simulink model "iot_casestudy_1_16"  (R2023a)
settings: Solver=VariableStepAuto  StartTime=0.0  StopTime=3.0  RelTol=1e-3
undefined symbols (not defined in the file or in its folder): m, n
(part 2 of 2)

== stateflow chart iot_casestudy_1_16/CameraDriver13 ==
  settings: updateMethod=CONTINUOUS
  state Operation
    state CarVisibility [parallel]
      settings: executionOrder=1
      state NoCar
        entry: car=0;
      state Car
        entry: car=1;
      (default) -> NoCar
      NoCar -> Car : [traffic_state==1]
      Car -> NoCar : [traffic_state==0]
    state DriverOperation [parallel]
      settings: executionOrder=2
      state Main
      (default) -> Main : {i=1;}
      Main -> (junction 22) : schedule
          | [image_request]
      (junction 22) -> Main [order 1] : [(car==1)&&(blurryness(i)==1)]
          | {image.data=1;send(image);i = i + 1;}
      (junction 22) -> Main [order 2] : {image.data=0;
          | send(image);i = i + 1;}
  data: image_request input; traffic_state input; blurryness input; image output; car local; i local; schedule input

== stateflow chart iot_casestudy_1_16/CameraDriver14 ==
  settings: updateMethod=CONTINUOUS
  state Operation
    state CarVisibility [parallel]
      settings: executionOrder=1
      state NoCar
        entry: car=0;
      state Car
        entry: car=1;
      (default) -> NoCar
      NoCar -> Car : [traffic_state==1]
      Car -> NoCar : [traffic_state==0]
    state DriverOperation [parallel]
      settings: executionOrder=2
      state Main
      (default) -> Main : {i=1;}
      Main -> (junction 22) : schedule[image_request]
      (junction 22) -> Main [order 2] : {image.data=0;
          | send(image);i = i + 1;}
      (junction 22) -> Main [order 1] : [(car==1)&&(blurryness(i)==1)]
          | {image.data=1;i = i + 1;send(image);}
  data: image_request input; traffic_state input; blurryness input; image output; car local; i local; schedule input

== stateflow chart iot_casestudy_1_16/CameraDriver15 ==
  settings: updateMethod=CONTINUOUS
  state Operation
    state CarVisibility [parallel]
      settings: executionOrder=1
      state NoCar
        entry: car=0;
      state Car
        entry: car=1;
      (default) -> NoCar
      NoCar -> Car : [traffic_state==1]
      Car -> NoCar : [traffic_state==0]
    state DriverOperation [parallel]
      settings: executionOrder=2
      state Main
      (default) -> Main : {i=1;}
      Main -> (junction 22) : schedule
          | [image_request]
      (junction 22) -> Main [order 1] : [(car==1)&&(blurryness(i)==1)]
          | {image.data=1;send(image);i = i + 1;}
      (junction 22) -> Main [order 2] : {image.data=0;
          | send(image);i = i + 1;}
  data: image_request input; traffic_state input; blurryness input; image output; car local; i local; schedule input

== stateflow chart iot_casestudy_1_16/CameraDriver8 ==
  settings: updateMethod=CONTINUOUS
  state Operation
    state CarVisibility [parallel]
      settings: executionOrder=1
      state NoCar
        entry: car=0;
      state Car
        entry: car=1;
      (default) -> NoCar
      NoCar -> Car : [traffic_state==1]
      Car -> NoCar : [traffic_state==0]
    state DriverOperation [parallel]
      settings: executionOrder=2
      state Main
      (default) -> Main : {i=1;}
      Main -> (junction 22) : schedule[image_request]
      (junction 22) -> Main [order 2] : {image.data=0;
          | send(image);i = i + 1;}
      (junction 22) -> Main [order 1] : [(car==1)&&(blurryness(i)==1)]
          | {image.data=1;i = i + 1;send(image);}
  data: image_request input; traffic_state input; blurryness input; image output; car local; i local; schedule input

== stateflow chart iot_casestudy_1_16/CameraDriver9 ==
  settings: updateMethod=CONTINUOUS
  state Operation
    state CarVisibility [parallel]
      settings: executionOrder=1
      state NoCar
        entry: car=0;
      state Car
        entry: car=1;
      (default) -> NoCar
      NoCar -> Car : [traffic_state==1]
      Car -> NoCar : [traffic_state==0]
    state DriverOperation [parallel]
      settings: executionOrder=2
      state Main
      (default) -> Main : {i=1;}
      Main -> (junction 22) : schedule
          | [image_request]
      (junction 22) -> Main [order 1] : [(car==1)&&(blurryness(i)==1)]
          | {image.data=1;send(image);i = i + 1;}
      (junction 22) -> Main [order 2] : {image.data=0;
          | send(image);i = i + 1;}
  data: image_request input; traffic_state input; blurryness input; image output; car local; i local; schedule input

== stateflow chart iot_casestudy_1_16/CameraScheduler10 ==
  settings: updateMethod=CONTINUOUS  executeAtInitialization=1
  state Main
    entry:
    dt=timer_array[i];
  (default) -> Main : {i=1;dt=0;}
  Main -> Main : after(dt,msec){i=i+1;send(schedule_driver);send(schedule_control);}
  data: timer_array input; schedule_driver output double; schedule_control output double; dt local double; dt2 local double; i local double =0.0

== stateflow chart iot_casestudy_1_16/CameraScheduler11 ==
  settings: updateMethod=CONTINUOUS  executeAtInitialization=1
  state Main
    entry:
    dt=timer_array[i];
  (default) -> Main : {i=0;dt=0;}
  Main -> Main : after(dt,msec){i=i+1;send(schedule_driver);send(schedule_control);}
  data: timer_array input; i local double; schedule_driver output double; schedule_control output double; dt local double

== stateflow chart iot_casestudy_1_16/CameraScheduler12 ==
  settings: updateMethod=CONTINUOUS  executeAtInitialization=1
  state Main
    entry:
    dt=timer_array[i];
  (default) -> Main : {i=1;dt=0;}
  Main -> Main : after(dt,msec){i=i+1;send(schedule_driver);send(schedule_control);}
  data: timer_array input; schedule_driver output double; schedule_control output double; dt local double; dt2 local double; i local double =0.0

== stateflow chart iot_casestudy_1_16/CameraScheduler13 ==
  settings: updateMethod=CONTINUOUS  executeAtInitialization=1
  state Main
    entry:
    dt=timer_array[i];
  (default) -> Main : {i=0;dt=0;}
  Main -> Main : after(dt,msec){i=i+1;send(schedule_driver);send(schedule_control);}
  data: timer_array input; i local double; schedule_driver output double; schedule_control output double; dt local double

== stateflow chart iot_casestudy_1_16/CameraScheduler14 ==
  settings: updateMethod=CONTINUOUS  executeAtInitialization=1
  state Main
    entry:
    dt=timer_array[i];
  (default) -> Main : {i=1;dt=0;}
  Main -> Main : after(dt,msec){i=i+1;send(schedule_driver);send(schedule_control);}
  data: timer_array input; schedule_driver output double; schedule_control output double; dt local double; dt2 local double; i local double =0.0

== stateflow chart iot_casestudy_1_16/CameraScheduler15 ==
  settings: updateMethod=CONTINUOUS  executeAtInitialization=1
  state Main
    entry:
    dt=timer_array[i];
  (default) -> Main : {i=0;dt=0;}
  Main -> Main : after(dt,msec){i=i+1;send(schedule_driver);send(schedule_control);}
  data: timer_array input; i local double; schedule_driver output double; schedule_control output double; dt local double

== stateflow chart iot_casestudy_1_16/CameraScheduler8 ==
  settings: updateMethod=CONTINUOUS  executeAtInitialization=1
  state Main
    entry:
    dt=timer_array[i];
  (default) -> Main : {i=1;dt=0;}
  Main -> Main : after(dt,msec){i=i+1;send(schedule_driver);send(schedule_control);}
  data: timer_array input; schedule_driver output double; schedule_control output double; dt local double; dt2 local double; i local double =0.0

== stateflow chart iot_casestudy_1_16/CameraScheduler9 ==
  settings: updateMethod=CONTINUOUS  executeAtInitialization=1
  state Main
    entry:
    dt=timer_array[i];
  (default) -> Main : {i=0;dt=0;}
  Main -> Main : after(dt,msec){i=i+1;send(schedule_driver);send(schedule_control);}
  data: timer_array input; i local double; schedule_driver output double; schedule_control output double; dt local double

== stateflow chart iot_casestudy_1_16/CameraDriver ==
  settings: updateMethod=CONTINUOUS
  state Operation
    state CarVisibility [parallel]
      settings: executionOrder=1
      state NoCar
        entry: car=0;
      state Car
        entry: car=1;
      (default) -> NoCar
      NoCar -> Car : [traffic_state==1]
      Car -> NoCar : [traffic_state==0]
    state DriverOperation [parallel]
      settings: executionOrder=2
      state Main
      (default) -> Main : {i=1;}
      Main -> (junction 22) : schedule[image_request]
      (junction 22) -> Main [order 2] : {image.data=0;
          | send(image);i = i + 1;}
      (junction 22) -> Main [order 1] : [(car==1)&&(blurryness(i)==1)]
          | {image.data=1;i = i + 1;send(image);}
  data: image_request input; traffic_state input; blurryness input; image output; car local; i local; schedule input

== stateflow chart iot_casestudy_1_16/CameraControl ==
  settings: updateMethod=CONTINUOUS
  state Operation
    state RequestHangling [parallel]
      settings: executionOrder=1
      state Operation1
      (default) -> Operation1 : {image_request=1;}
      Operation1 -> Operation1 : schedule{image_request=1;}
    state ImageMessaging [parallel]
      settings: executionOrder=2
      state Operation2
        entry:
        validity=isvalid(imageIn);
      (default) -> Operation2 : {i=1;}
      (junction 28) -> Operation2 [order 1] : [validity==1]
          | {receive(imageIn);i = i + 1;
          | imageOut.data=imageIn.data
          | send(imageOut);}
      (junction 28) -> Operation2 [order 2] : {i = i + 1;receive(imageIn);}
      (junction 19) -> (junction 28) [order 1] : [network_faults(i)==0]
      (junction 19) -> Operation2 [order 2] : {receive(imageIn);i = i + 1;}
      Operation2 -> (junction 19) : schedule
  (default) -> Operation
  data: image_request output; imageIn input; i local; network_faults input; imageOut output; schedule input; validity local

== stateflow chart iot_casestudy_1_16/Traffic ==
  settings: updateMethod=CONTINUOUS
  state Nocar
    entry:
    traffic_state=0;
  state Car
    entry:
    traffic_state=1;
  state Nocar1
    entry:
    traffic_state=0;
  (default) -> Nocar
  Nocar -> Car : after(arrive_time,msec)
  Car -> Nocar1 : after(visibility_time,msec)
  data: arrive_time input; visibility_time input; traffic_state output

== stateflow chart iot_casestudy_1_16/Edge ==
  state Waiting
  state NotRecognized
    wait_time=elapsed(msec);
  state Recognized
  (default) -> Waiting : {faults=0;}
  Waiting -> Waiting [order 2] : image2{receive(image2);}
  Waiting -> Waiting [order 7] : image5{receive(image5);}
  Waiting -> Waiting [order 8] : image7{receive(image7);}
  Waiting -> Waiting [order 5] : image3{receive(image3);}
  Waiting -> Waiting [order 9] : image8{receive(image8);}
  Waiting -> Waiting [order 6] : image4{receive(image4);}
  Waiting -> Waiting [order 3] : image1{receive(image1);}
  Waiting -> Waiting [order 1] : image6{receive(image6);}
  Waiting -> NotRecognized [order 4] : [traffic_state==1]
  NotRecognized -> Waiting [order 1] : [traffic_state==0]
      | {faults=1;}
  Recognized -> Waiting [order 1] : [traffic_state==0]
  Waiting -> Waiting [order 10] : image9{receive(image9);}
  Waiting -> Waiting [order 11] : image10{receive(image10);}
  Waiting -> Waiting [order 12] : image11{receive(image11);}
  Waiting -> Waiting [order 13] : image12{receive(image12);}
  Waiting -> Waiting [order 14] : image13{receive(image13);}
  Waiting -> Waiting [order 15] : image14{receive(image14);}
  Waiting -> Waiting [order 16] : image15{receive(image15);}
  Waiting -> Waiting [order 17] : image16{receive(image16);}
  (junction 119) -> NotRecognized [order 2]
  NotRecognized -> (junction 119) [order 3] : image16
      | {receive(image16);}
  (junction 117) -> NotRecognized [order 2]
  NotRecognized -> (junction 117) [order 4] : image15
      | {receive(image15);}
  (junction 106) -> NotRecognized [order 2]
  NotRecognized -> (junction 106) [order 5] : image14
      | {receive(image14);}
  (junction 132) -> NotRecognized [order 2]
  NotRecognized -> (junction 132) [order 6] : image13
      | {receive(image13);}
  (junction 108) -> NotRecognized [order 2]
  NotRecognized -> (junction 108) [order 7] : image12
      | {receive(image12);}
  (junction 113) -> NotRecognized [order 2]
  NotRecognized -> (junction 113) [order 8] : image11
      | {receive(image11);}
  (junction 105) -> NotRecognized [order 2]
  NotRecognized -> (junction 105) [order 9] : image10
      | {receive(image10);}
  (junction 120) -> NotRecognized [order 2]
  NotRecognized -> (junction 120) [order 11] : image9
      | {receive(image9);}
  (junction 64) -> NotRecognized [order 2]
  NotRecognized -> (junction 64) [order 17] : image8
      | {receive(image8);}
  (junction 63) -> NotRecognized [order 2]
  NotRecognized -> (junction 63) [order 16] : image7
      | {receive(image7);}
  (junction 62) -> NotRecognized [order 2]
  NotRecognized -> (junction 62) [order 15] : image6
      | {receive(image6);}
  (junction 61) -> NotRecognized [order 2]
  NotRecognized -> (junction 61) [order 14] : image5
      | {receive(image5);}
  (junction 49) -> NotRecognized [order 2]
  NotRecognized -> (junction 49) [order 13] : image4
      | {receive(image4);}
  (junction 45) -> NotRecognized [order 2]
  NotRecognized -> (junction 45) [order 12] : image3
      | {receive(image3);}
  (junction 22) -> NotRecognized [order 2]
  NotRecognized -> (junction 22) [order 2] : image2
      | {receive(image2);}
  (junction 10) -> NotRecognized [order 2]
  NotRecognized -> (junction 10) [order 10] : image1{receive(image1);}
  (junction 49) -> Recognized [order 1] : [image4.data==1]
  (junction 22) -> Recognized [order 1] : [image2.data==1]
  (junction 105) -> Recognized [order 1] : [image10.data==1]
  (junction 64) -> Recognized [order 1] : [image8.data==1]
  (junction 62) -> Recognized [order 1] : [image6.data==1]
  (junction 119) -> Recognized [order 1] : [image16.data==1]
  (junction 106) -> Recognized [order 1] : [image14.data==1]
  (junction 108) -> Recognized [order 1] : [image12.data==1]
  (junction 132) -> Recognized [order 1] : [image13.data==1]
  (junction 113) -> Recognized [order 1] : [image11.data==1]
  (junction 120) -> Recognized [order 1] : [image9.data==1]
  (junction 63) -> Recognized [order 1] : [image7.data==1]
  (junction 61) -> Recognized [order 1] : [image5.data==1]
  (junction 117) -> Recognized [order 1] : [image15.data==1]
  (junction 45) -> Recognized [order 1] : [image3.data==1]
  (junction 10) -> Recognized [order 1] : [image1.data==1]
  Recognized -> Recognized [order 10] : image9{receive(image9);}
  Recognized -> Recognized [order 11] : image10{receive(image10);}
  Recognized -> Recognized [order 12] : image11{receive(image11);}
  Recognized -> Recognized [order 13] : image12{receive(image12);}
  Recognized -> Recognized [order 14] : image13{receive(image13);}
  Recognized -> Recognized [order 15] : image14{receive(image14);}
  Recognized -> Recognized [order 16] : image15{receive(image15);}
  Recognized -> Recognized [order 17] : image16{receive(image16);}
  Recognized -> Recognized [order 6] : image8{receive(image8);}
  Recognized -> Recognized [order 7] : image7{receive(image7);}
  Recognized -> Recognized [order 8] : image6{receive(image6);}
  Recognized -> Recognized [order 9] : image5{receive(image5);}
  Recognized -> Recognized [order 2] : image3{receive(image3);}
  Recognized -> Recognized [order 5] : image4{receive(image4);}
  Recognized -> Recognized [order 3] : image2{receive(image2);}
  Recognized -> Recognized [order 4] : image1{receive(image1);}
  data: traffic_state input; image1 input; faults output; image2 input; wait_time output; image3 input; image4 input; image5 input; image6 input; image7 input; image8 input; image9 input; image10 input; image11 input; image12 input; image13 input; image14 input; image15 input; image16 input

== stateflow chart iot_casestudy_1_16/CameraScheduler ==
  settings: updateMethod=CONTINUOUS  executeAtInitialization=1
  state Main
    entry:
    dt=timer_array[i];
  (default) -> Main : {i=1;dt=0;}
  Main -> Main : after(dt,msec){i=i+1;send(schedule_driver);send(schedule_control);}
  data: timer_array input; schedule_driver output double; schedule_control output double; dt local double; dt2 local double; i output double =0.0

== stateflow chart iot_casestudy_1_16/CameraControl1 ==
  settings: updateMethod=CONTINUOUS
  state Operation
    state RequestHangling [parallel]
      settings: executionOrder=1
      note: {image_request=1;}
      state Operation1
      (default) -> Operation1
      Operation1 -> Operation1 : schedule{image_request=1;}
    state ImageMessaging [parallel]
      settings: executionOrder=2
      state Operation2
        entry:
        validity=isvalid(imageIn);
      (default) -> Operation2 : {i=1;}
      (junction 29) -> Operation2 [order 1] : [isvalid(imageIn)==1]
          | {receive(imageIn);i = i + 1;
          | imageOut.data=imageIn.data;
          | send(imageOut);}
      (junction 19) -> Operation2 [order 2] : {receive(imageIn);i = i + 1;}
      Operation2 -> (junction 19) : schedule
      (junction 29) -> Operation2 [order 2] : {i = i + 1;receive(imageIn);}
      (junction 19) -> (junction 29) [order 1] : [network_faults(i)==0]
  (default) -> Operation
  data: image_request output; imageIn input; i local; network_faults input; imageOut output; schedule input; validity local

== stateflow chart iot_casestudy_1_16/CameraDriver1 ==
  settings: updateMethod=CONTINUOUS
  state Operation
    state CarVisibility [parallel]
      settings: executionOrder=1
      state NoCar
        entry: car=0;
      state Car
        entry: car=1;
      (default) -> NoCar
      NoCar -> Car : [traffic_state==1]
      Car -> NoCar : [traffic_state==0]
    state DriverOperation [parallel]
      settings: executionOrder=2
      state Main
      (default) -> Main : {i=1;}
      Main -> (junction 22) : schedule
          | [image_request]
      (junction 22) -> Main [order 1] : [(car==1)&&(blurryness(i)==1)]
          | {image.data=1;send(image);i = i + 1;}
      (junction 22) -> Main [order 2] : {image.data=0;
          | send(image);i = i + 1;}
  data: image_request input; traffic_state input; blurryness input; image output; car local; i local; schedule input

== stateflow chart iot_casestudy_1_16/CameraScheduler1 ==
  settings: updateMethod=CONTINUOUS  executeAtInitialization=1
  state Main
    entry:
    dt=timer_array[i];
  (default) -> Main : {i=0;dt=0;}
  Main -> Main : after(dt,msec){i=i+1;send(schedule_driver);send(schedule_control);}
  data: timer_array input; i local double; schedule_driver output double; schedule_control output double; dt local double

== stateflow chart iot_casestudy_1_16/CameraControl2 ==
  settings: updateMethod=CONTINUOUS
  state Operation
    state RequestHangling [parallel]
      settings: executionOrder=1
      state Operation1
      (default) -> Operation1 : {image_request=1;}
      Operation1 -> Operation1 : schedule{image_request=1;}
    state ImageMessaging [parallel]
      settings: executionOrder=2
      state Operation2
        entry:
        validity=isvalid(imageIn);
      (default) -> Operation2 : {i=1;}
      (junction 28) -> Operation2 [order 1] : [validity==1]
          | {receive(imageIn);i = i + 1;
          | imageOut.data=imageIn.data
          | send(imageOut);}
      (junction 28) -> Operation2 [order 2] : {i = i + 1;receive(imageIn);}
      (junction 19) -> (junction 28) [order 1] : [network_faults(i)==0]
      (junction 19) -> Operation2 [order 2] : {receive(imageIn);i = i + 1;}
      Operation2 -> (junction 19) : schedule
  (default) -> Operation
  data: image_request output; imageIn input; i local; network_faults input; imageOut output; schedule input; validity local

== stateflow chart iot_casestudy_1_16/CameraControl3 ==
  settings: updateMethod=CONTINUOUS
  state Operation
    state RequestHangling [parallel]
      settings: executionOrder=1
      note: {image_request=1;}
      state Operation1
      (default) -> Operation1
      Operation1 -> Operation1 : schedule{image_request=1;}
    state ImageMessaging [parallel]
      settings: executionOrder=2
      state Operation2
        entry:
        validity=isvalid(imageIn);
      (default) -> Operation2 : {i=1;}
      (junction 29) -> Operation2 [order 1] : [isvalid(imageIn)==1]
          | {receive(imageIn);i = i + 1;
          | imageOut.data=imageIn.data;
          | send(imageOut);}
      (junction 19) -> Operation2 [order 2] : {receive(imageIn);i = i + 1;}
      Operation2 -> (junction 19) : schedule
      (junction 29) -> Operation2 [order 2] : {i = i + 1;receive(imageIn);}
      (junction 19) -> (junction 29) [order 1] : [network_faults(i)==0]
  (default) -> Operation
  data: image_request output; imageIn input; i local; network_faults input; imageOut output; schedule input; validity local

== stateflow chart iot_casestudy_1_16/CameraDriver2 ==
  settings: updateMethod=CONTINUOUS
  state Operation
    state CarVisibility [parallel]
      settings: executionOrder=1
      state NoCar
        entry: car=0;
      state Car
        entry: car=1;
      (default) -> NoCar
      NoCar -> Car : [traffic_state==1]
      Car -> NoCar : [traffic_state==0]
    state DriverOperation [parallel]
      settings: executionOrder=2
      state Main
      (default) -> Main : {i=1;}
      Main -> (junction 22) : schedule[image_request]
      (junction 22) -> Main [order 2] : {image.data=0;
          | send(image);i = i + 1;}
      (junction 22) -> Main [order 1] : [(car==1)&&(blurryness(i)==1)]
          | {image.data=1;i = i + 1;send(image);}
  data: image_request input; traffic_state input; blurryness input; image output; car local; i local; schedule input

== stateflow chart iot_casestudy_1_16/CameraDriver3 ==
  settings: updateMethod=CONTINUOUS
  state Operation
    state CarVisibility [parallel]
      settings: executionOrder=1
      state NoCar
        entry: car=0;
      state Car
        entry: car=1;
      (default) -> NoCar
      NoCar -> Car : [traffic_state==1]
      Car -> NoCar : [traffic_state==0]
    state DriverOperation [parallel]
      settings: executionOrder=2
      state Main
      (default) -> Main : {i=1;}
      Main -> (junction 22) : schedule
          | [image_request]
      (junction 22) -> Main [order 1] : [(car==1)&&(blurryness(i)==1)]
          | {image.data=1;send(image);i = i + 1;}
      (junction 22) -> Main [order 2] : {image.data=0;
          | send(image);i = i + 1;}
  data: image_request input; traffic_state input; blurryness input; image output; car local; i local; schedule input

== stateflow chart iot_casestudy_1_16/CameraScheduler2 ==
  settings: updateMethod=CONTINUOUS  executeAtInitialization=1
  state Main
    entry:
    dt=timer_array[i];
  (default) -> Main : {i=1;dt=0;}
  Main -> Main : after(dt,msec){i=i+1;send(schedule_driver);send(schedule_control);}
  data: timer_array input; schedule_driver output double; schedule_control output double; dt local double; dt2 local double; i output double =0.0

== stateflow chart iot_casestudy_1_16/CameraScheduler3 ==
  settings: updateMethod=CONTINUOUS  executeAtInitialization=1
  state Main
    entry:
    dt=timer_array[i];
  (default) -> Main : {i=0;dt=0;}
  Main -> Main : after(dt,msec){i=i+1;send(schedule_driver);send(schedule_control);}
  data: timer_array input; i local double; schedule_driver output double; schedule_control output double; dt local double

== stateflow chart iot_casestudy_1_16/CameraControl4 ==
  settings: updateMethod=CONTINUOUS
  state Operation
    state RequestHangling [parallel]
      settings: executionOrder=1
      state Operation1
      (default) -> Operation1 : {image_request=1;}
      Operation1 -> Operation1 : schedule{image_request=1;}
    state ImageMessaging [parallel]
      settings: executionOrder=2
      state Operation2
        entry:
        validity=isvalid(imageIn);
      (default) -> Operation2 : {i=1;}
      (junction 28) -> Operation2 [order 1] : [validity==1]
          | {receive(imageIn);i = i + 1;
          | imageOut.data=imageIn.data
          | send(imageOut);}
      (junction 28) -> Operation2 [order 2] : {i = i + 1;receive(imageIn);}
      (junction 19) -> (junction 28) [order 1] : [network_faults(i)==0]
      (junction 19) -> Operation2 [order 2] : {receive(imageIn);i = i + 1;}
      Operation2 -> (junction 19) : schedule
  (default) -> Operation
  data: image_request output; imageIn input; i local; network_faults input; imageOut output; schedule input; validity local

== stateflow chart iot_casestudy_1_16/CameraControl5 ==
  settings: updateMethod=CONTINUOUS
  state Operation
    state RequestHangling [parallel]
      settings: executionOrder=1
      note: {image_request=1;}
      state Operation1
      (default) -> Operation1
      Operation1 -> Operation1 : schedule{image_request=1;}
    state ImageMessaging [parallel]
      settings: executionOrder=2
      state Operation2
        entry:
        validity=isvalid(imageIn);
      (default) -> Operation2 : {i=1;}
      (junction 29) -> Operation2 [order 1] : [isvalid(imageIn)==1]
          | {receive(imageIn);i = i + 1;
          | imageOut.data=imageIn.data;
          | send(imageOut);}
      (junction 19) -> Operation2 [order 2] : {receive(imageIn);i = i + 1;}
      Operation2 -> (junction 19) : schedule
      (junction 29) -> Operation2 [order 2] : {i = i + 1;receive(imageIn);}
      (junction 19) -> (junction 29) [order 1] : [network_faults(i)==0]
  (default) -> Operation
  data: image_request output; imageIn input; i local; network_faults input; imageOut output; schedule input; validity local

== stateflow chart iot_casestudy_1_16/CameraControl6 ==
  settings: updateMethod=CONTINUOUS
  state Operation
    state RequestHangling [parallel]
      settings: executionOrder=1
      state Operation1
      (default) -> Operation1 : {image_request=1;}
      Operation1 -> Operation1 : schedule{image_request=1;}
    state ImageMessaging [parallel]
      settings: executionOrder=2
      state Operation2
        entry:
        validity=isvalid(imageIn);
      (default) -> Operation2 : {i=1;}
      (junction 28) -> Operation2 [order 1] : [validity==1]
          | {receive(imageIn);i = i + 1;
          | imageOut.data=imageIn.data
          | send(imageOut);}
      (junction 28) -> Operation2 [order 2] : {i = i + 1;receive(imageIn);}
      (junction 19) -> (junction 28) [order 1] : [network_faults(i)==0]
      (junction 19) -> Operation2 [order 2] : {receive(imageIn);i = i + 1;}
      Operation2 -> (junction 19) : schedule
  (default) -> Operation
  data: image_request output; imageIn input; i local; network_faults input; imageOut output; schedule input; validity local

== stateflow chart iot_casestudy_1_16/CameraControl7 ==
  settings: updateMethod=CONTINUOUS
  state Operation
    state RequestHangling [parallel]
      settings: executionOrder=1
      note: {image_request=1;}
      state Operation1
      (default) -> Operation1
      Operation1 -> Operation1 : schedule{image_request=1;}
    state ImageMessaging [parallel]
      settings: executionOrder=2
      state Operation2
        entry:
        validity=isvalid(imageIn);
      (default) -> Operation2 : {i=1;}
      (junction 29) -> Operation2 [order 1] : [isvalid(imageIn)==1]
          | {receive(imageIn);i = i + 1;
          | imageOut.data=imageIn.data;
          | send(imageOut);}
      (junction 19) -> Operation2 [order 2] : {receive(imageIn);i = i + 1;}
      Operation2 -> (junction 19) : schedule
      (junction 29) -> Operation2 [order 2] : {i = i + 1;receive(imageIn);}
      (junction 19) -> (junction 29) [order 1] : [network_faults(i)==0]
  (default) -> Operation
  data: image_request output; imageIn input; i local; network_faults input; imageOut output; schedule input; validity local

== stateflow chart iot_casestudy_1_16/CameraDriver4 ==
  settings: updateMethod=CONTINUOUS
  state Operation
    state CarVisibility [parallel]
      settings: executionOrder=1
      state NoCar
        entry: car=0;
      state Car
        entry: car=1;
      (default) -> NoCar
      NoCar -> Car : [traffic_state==1]
      Car -> NoCar : [traffic_state==0]
    state DriverOperation [parallel]
      settings: executionOrder=2
      state Main
      (default) -> Main : {i=1;}
      Main -> (junction 22) : schedule[image_request]
      (junction 22) -> Main [order 2] : {image.data=0;
          | send(image);i = i + 1;}
      (junction 22) -> Main [order 1] : [(car==1)&&(blurryness(i)==1)]
          | {image.data=1;i = i + 1;send(image);}
  data: image_request input; traffic_state input; blurryness input; image output; car local; i local; schedule input

== stateflow chart iot_casestudy_1_16/CameraDriver5 ==
  settings: updateMethod=CONTINUOUS
  state Operation
    state CarVisibility [parallel]
      settings: executionOrder=1
      state NoCar
        entry: car=0;
      state Car
        entry: car=1;
      (default) -> NoCar
      NoCar -> Car : [traffic_state==1]
      Car -> NoCar : [traffic_state==0]
    state DriverOperation [parallel]
      settings: executionOrder=2
      state Main
      (default) -> Main : {i=1;}
      Main -> (junction 22) : schedule
          | [image_request]
      (junction 22) -> Main [order 1] : [(car==1)&&(blurryness(i)==1)]
          | {image.data=1;send(image);i = i + 1;}
      (junction 22) -> Main [order 2] : {image.data=0;
          | send(image);i = i + 1;}
  data: image_request input; traffic_state input; blurryness input; image output; car local; i local; schedule input

== stateflow chart iot_casestudy_1_16/CameraDriver6 ==
  settings: updateMethod=CONTINUOUS
  state Operation
    state CarVisibility [parallel]
      settings: executionOrder=1
      state NoCar
        entry: car=0;
      state Car
        entry: car=1;
      (default) -> NoCar
      NoCar -> Car : [traffic_state==1]
      Car -> NoCar : [traffic_state==0]
    state DriverOperation [parallel]
      settings: executionOrder=2
      state Main
      (default) -> Main : {i=1;}
      Main -> (junction 22) : schedule[image_request]
      (junction 22) -> Main [order 2] : {image.data=0;
          | send(image);i = i + 1;}
      (junction 22) -> Main [order 1] : [(car==1)&&(blurryness(i)==1)]
          | {image.data=1;i = i + 1;send(image);}
  data: image_request input; traffic_state input; blurryness input; image output; car local; i local; schedule input

== stateflow chart iot_casestudy_1_16/CameraDriver7 ==
  settings: updateMethod=CONTINUOUS
  state Operation
    state CarVisibility [parallel]
      settings: executionOrder=1
      state NoCar
        entry: car=0;
      state Car
        entry: car=1;
      (default) -> NoCar
      NoCar -> Car : [traffic_state==1]
      Car -> NoCar : [traffic_state==0]
    state DriverOperation [parallel]
      settings: executionOrder=2
      state Main
      (default) -> Main : {i=1;}
      Main -> (junction 22) : schedule
          | [image_request]
      (junction 22) -> Main [order 1] : [(car==1)&&(blurryness(i)==1)]
          | {image.data=1;send(image);i = i + 1;}
      (junction 22) -> Main [order 2] : {image.data=0;
          | send(image);i = i + 1;}
  data: image_request input; traffic_state input; blurryness input; image output; car local; i local; schedule input

== stateflow chart iot_casestudy_1_16/CameraScheduler4 ==
  settings: updateMethod=CONTINUOUS  executeAtInitialization=1
  state Main
    entry:
    dt=timer_array[i];
  (default) -> Main : {i=1;dt=0;}
  Main -> Main : after(dt,msec){i=i+1;send(schedule_driver);send(schedule_control);}
  data: timer_array input; schedule_driver output double; schedule_control output double; dt local double; dt2 local double; i output double =0.0

== stateflow chart iot_casestudy_1_16/CameraScheduler5 ==
  settings: updateMethod=CONTINUOUS  executeAtInitialization=1
  state Main
    entry:
    dt=timer_array[i];
  (default) -> Main : {i=0;dt=0;}
  Main -> Main : after(dt,msec){i=i+1;send(schedule_driver);send(schedule_control);}
  data: timer_array input; i local double; schedule_driver output double; schedule_control output double; dt local double

== stateflow chart iot_casestudy_1_16/CameraScheduler6 ==
  settings: updateMethod=CONTINUOUS  executeAtInitialization=1
  state Main
    entry:
    dt=timer_array[i];
  (default) -> Main : {i=1;dt=0;}
  Main -> Main : after(dt,msec){i=i+1;send(schedule_driver);send(schedule_control);}
  data: timer_array input; schedule_driver output double; schedule_control output double; dt local double; dt2 local double; i output double =0.0

== stateflow chart iot_casestudy_1_16/CameraScheduler7 ==
  settings: updateMethod=CONTINUOUS  executeAtInitialization=1
  state Main
    entry:
    dt=timer_array[i];
  (default) -> Main : {i=0;dt=0;}
  Main -> Main : after(dt,msec){i=i+1;send(schedule_driver);send(schedule_control);}
  data: timer_array input; i local double; schedule_driver output double; schedule_control output double; dt local double

== stateflow chart iot_casestudy_1_16/CameraControl10 ==
  settings: updateMethod=CONTINUOUS
  state Operation
    state RequestHangling [parallel]
      settings: executionOrder=1
      state Operation1
      (default) -> Operation1 : {image_request=1;}
      Operation1 -> Operation1 : schedule{image_request=1;}
    state ImageMessaging [parallel]
      settings: executionOrder=2
      state Operation2
        entry:
        validity=isvalid(imageIn);
      (default) -> Operation2 : {i=1;}
      (junction 28) -> Operation2 [order 1] : [validity==1]
          | {receive(imageIn);i = i + 1;
          | imageOut.data=imageIn.data
          | send(imageOut);}
      (junction 28) -> Operation2 [order 2] : {i = i + 1;receive(imageIn);}
      (junction 19) -> (junction 28) [order 1] : [network_faults(i)==0]
      (junction 19) -> Operation2 [order 2] : {receive(imageIn);i = i + 1;}
      Operation2 -> (junction 19) : schedule
  (default) -> Operation
  data: image_request output; imageIn input; i local; network_faults input; imageOut output; schedule input; validity local

== stateflow chart iot_casestudy_1_16/CameraControl11 ==
  settings: updateMethod=CONTINUOUS
  state Operation
    state RequestHangling [parallel]
      settings: executionOrder=1
      note: {image_request=1;}
      state Operation1
      (default) -> Operation1
      Operation1 -> Operation1 : schedule{image_request=1;}
    state ImageMessaging [parallel]
      settings: executionOrder=2
      state Operation2
        entry:
        validity=isvalid(imageIn);
      (default) -> Operation2 : {i=1;}
      (junction 29) -> Operation2 [order 1] : [isvalid(imageIn)==1]
          | {receive(imageIn);i = i + 1;
          | imageOut.data=imageIn.data;
          | send(imageOut);}
      (junction 19) -> Operation2 [order 2] : {receive(imageIn);i = i + 1;}
      Operation2 -> (junction 19) : schedule
      (junction 29) -> Operation2 [order 2] : {i = i + 1;receive(imageIn);}
      (junction 19) -> (junction 29) [order 1] : [network_faults(i)==0]
  (default) -> Operation
  data: image_request output; imageIn input; i local; network_faults input; imageOut output; schedule input; validity local

== stateflow chart iot_casestudy_1_16/CameraControl12 ==
  settings: updateMethod=CONTINUOUS
  state Operation
    state RequestHangling [parallel]
      settings: executionOrder=1
      state Operation1
      (default) -> Operation1 : {image_request=1;}
      Operation1 -> Operation1 : schedule{image_request=1;}
    state ImageMessaging [parallel]
      settings: executionOrder=2
      state Operation2
        entry:
        validity=isvalid(imageIn);
      (default) -> Operation2 : {i=1;}
      (junction 28) -> Operation2 [order 1] : [validity==1]
          | {receive(imageIn);i = i + 1;
          | imageOut.data=imageIn.data
          | send(imageOut);}
      (junction 28) -> Operation2 [order 2] : {i = i + 1;receive(imageIn);}
      (junction 19) -> (junction 28) [order 1] : [network_faults(i)==0]
      (junction 19) -> Operation2 [order 2] : {receive(imageIn);i = i + 1;}
      Operation2 -> (junction 19) : schedule
  (default) -> Operation
  data: image_request output; imageIn input; i local; network_faults input; imageOut output; schedule input; validity local

== stateflow chart iot_casestudy_1_16/CameraControl13 ==
  settings: updateMethod=CONTINUOUS
  state Operation
    state RequestHangling [parallel]
      settings: executionOrder=1
      note: {image_request=1;}
      state Operation1
      (default) -> Operation1
      Operation1 -> Operation1 : schedule{image_request=1;}
    state ImageMessaging [parallel]
      settings: executionOrder=2
      state Operation2
        entry:
        validity=isvalid(imageIn);
      (default) -> Operation2 : {i=1;}
      (junction 29) -> Operation2 [order 1] : [isvalid(imageIn)==1]
          | {receive(imageIn);i = i + 1;
          | imageOut.data=imageIn.data;
          | send(imageOut);}
      (junction 19) -> Operation2 [order 2] : {receive(imageIn);i = i + 1;}
      Operation2 -> (junction 19) : schedule
      (junction 29) -> Operation2 [order 2] : {i = i + 1;receive(imageIn);}
      (junction 19) -> (junction 29) [order 1] : [network_faults(i)==0]
  (default) -> Operation
  data: image_request output; imageIn input; i local; network_faults input; imageOut output; schedule input; validity local

== stateflow chart iot_casestudy_1_16/CameraControl14 ==
  settings: updateMethod=CONTINUOUS
  state Operation
    state RequestHangling [parallel]
      settings: executionOrder=1
      state Operation1
      (default) -> Operation1 : {image_request=1;}
      Operation1 -> Operation1 : schedule{image_request=1;}
    state ImageMessaging [parallel]
      settings: executionOrder=2
      state Operation2
        entry:
        validity=isvalid(imageIn);
      (default) -> Operation2 : {i=1;}
      (junction 28) -> Operation2 [order 1] : [validity==1]
          | {receive(imageIn);i = i + 1;
          | imageOut.data=imageIn.data
          | send(imageOut);}
      (junction 28) -> Operation2 [order 2] : {i = i + 1;receive(imageIn);}
      (junction 19) -> (junction 28) [order 1] : [network_faults(i)==0]
      (junction 19) -> Operation2 [order 2] : {receive(imageIn);i = i + 1;}
      Operation2 -> (junction 19) : schedule
  (default) -> Operation
  data: image_request output; imageIn input; i local; network_faults input; imageOut output; schedule input; validity local

== stateflow chart iot_casestudy_1_16/CameraControl15 ==
  settings: updateMethod=CONTINUOUS
  state Operation
    state RequestHangling [parallel]
      settings: executionOrder=1
      note: {image_request=1;}
      state Operation1
      (default) -> Operation1
      Operation1 -> Operation1 : schedule{image_request=1;}
    state ImageMessaging [parallel]
      settings: executionOrder=2
      state Operation2
        entry:
        validity=isvalid(imageIn);
      (default) -> Operation2 : {i=1;}
      (junction 29) -> Operation2 [order 1] : [isvalid(imageIn)==1]
          | {receive(imageIn);i = i + 1;
          | imageOut.data=imageIn.data;
          | send(imageOut);}
      (junction 19) -> Operation2 [order 2] : {receive(imageIn);i = i + 1;}
      Operation2 -> (junction 19) : schedule
      (junction 29) -> Operation2 [order 2] : {i = i + 1;receive(imageIn);}
      (junction 19) -> (junction 29) [order 1] : [network_faults(i)==0]
  (default) -> Operation
  data: image_request output; imageIn input; i local; network_faults input; imageOut output; schedule input; validity local

== stateflow chart iot_casestudy_1_16/CameraControl8 ==
  settings: updateMethod=CONTINUOUS
  state Operation
    state RequestHangling [parallel]
      settings: executionOrder=1
      state Operation1
      (default) -> Operation1 : {image_request=1;}
      Operation1 -> Operation1 : schedule{image_request=1;}
    state ImageMessaging [parallel]
      settings: executionOrder=2
      state Operation2
        entry:
        validity=isvalid(imageIn);
      (default) -> Operation2 : {i=1;}
      (junction 28) -> Operation2 [order 1] : [validity==1]
          | {receive(imageIn);i = i + 1;
          | imageOut.data=imageIn.data
          | send(imageOut);}
      (junction 28) -> Operation2 [order 2] : {i = i + 1;receive(imageIn);}
      (junction 19) -> (junction 28) [order 1] : [network_faults(i)==0]
      (junction 19) -> Operation2 [order 2] : {receive(imageIn);i = i + 1;}
      Operation2 -> (junction 19) : schedule
  (default) -> Operation
  data: image_request output; imageIn input; i local; network_faults input; imageOut output; schedule input; validity local

== stateflow chart iot_casestudy_1_16/CameraControl9 ==
  settings: updateMethod=CONTINUOUS
  state Operation
    state RequestHangling [parallel]
      settings: executionOrder=1
      note: {image_request=1;}
      state Operation1
      (default) -> Operation1
      Operation1 -> Operation1 : schedule{image_request=1;}
    state ImageMessaging [parallel]
      settings: executionOrder=2
      state Operation2
        entry:
        validity=isvalid(imageIn);
      (default) -> Operation2 : {i=1;}
      (junction 29) -> Operation2 [order 1] : [isvalid(imageIn)==1]
          | {receive(imageIn);i = i + 1;
          | imageOut.data=imageIn.data;
          | send(imageOut);}
      (junction 19) -> Operation2 [order 2] : {receive(imageIn);i = i + 1;}
      Operation2 -> (junction 19) : schedule
      (junction 29) -> Operation2 [order 2] : {i = i + 1;receive(imageIn);}
      (junction 19) -> (junction 29) [order 1] : [network_faults(i)==0]
  (default) -> Operation
  data: image_request output; imageIn input; i local; network_faults input; imageOut output; schedule input; validity local

== stateflow chart iot_casestudy_1_16/CameraDriver10 ==
  settings: updateMethod=CONTINUOUS
  state Operation
    state CarVisibility [parallel]
      settings: executionOrder=1
      state NoCar
        entry: car=0;
      state Car
        entry: car=1;
      (default) -> NoCar
      NoCar -> Car : [traffic_state==1]
      Car -> NoCar : [traffic_state==0]
    state DriverOperation [parallel]
      settings: executionOrder=2
      state Main
      (default) -> Main : {i=1;}
      Main -> (junction 22) : schedule[image_request]
      (junction 22) -> Main [order 2] : {image.data=0;
          | send(image);i = i + 1;}
      (junction 22) -> Main [order 1] : [(car==1)&&(blurryness(i)==1)]
          | {image.data=1;i = i + 1;send(image);}
  data: image_request input; traffic_state input; blurryness input; image output; car local; i local; schedule input

== stateflow chart iot_casestudy_1_16/CameraDriver11 ==
  settings: updateMethod=CONTINUOUS
  state Operation
    state CarVisibility [parallel]
      settings: executionOrder=1
      state NoCar
        entry: car=0;
      state Car
        entry: car=1;
      (default) -> NoCar
      NoCar -> Car : [traffic_state==1]
      Car -> NoCar : [traffic_state==0]
    state DriverOperation [parallel]
      settings: executionOrder=2
      state Main
      (default) -> Main : {i=1;}
      Main -> (junction 22) : schedule
          | [image_request]
      (junction 22) -> Main [order 1] : [(car==1)&&(blurryness(i)==1)]
          | {image.data=1;send(image);i = i + 1;}
      (junction 22) -> Main [order 2] : {image.data=0;
          | send(image);i = i + 1;}
  data: image_request input; traffic_state input; blurryness input; image output; car local; i local; schedule input

== stateflow chart iot_casestudy_1_16/CameraDriver12 ==
  settings: updateMethod=CONTINUOUS
  state Operation
    state CarVisibility [parallel]
      settings: executionOrder=1
      state NoCar
        entry: car=0;
      state Car
        entry: car=1;
      (default) -> NoCar
      NoCar -> Car : [traffic_state==1]
      Car -> NoCar : [traffic_state==0]
    state DriverOperation [parallel]
      settings: executionOrder=2
      state Main
      (default) -> Main : {i=1;}
      Main -> (junction 22) : schedule[image_request]
      (junction 22) -> Main [order 2] : {image.data=0;
          | send(image);i = i + 1;}
      (junction 22) -> Main [order 1] : [(car==1)&&(blurryness(i)==1)]
          | {image.data=1;i = i + 1;send(image);}
  data: image_request input; traffic_state input; blurryness input; image output; car local; i local; schedule input
